simulink model "ProgrammablePulseGenerator"  (Simulink 7.8)
settings: Solver=FixedStepDiscrete  StartTime=0.0  StopTime=10  FixedStep=0.0001  RelTol=1e-3
PostLoadFcn:
  | , if any(exist('dsrtsu_mdlpostloadfcn', 'file') == [2, 3, 6]), try dsrtsu_mdlpostloadfcn('Execute', bdroot); catch fprintf('Error in PostLoadFcn (dsrtsu_mdlpostloadfcn) for model "%s":\n %s\n', bdroot, lasterr); end, end,
settings Model: DSRTSU_INTERNAL_RTI_VER=360  DSRTSU_INTERNAL_RTI_TYPE=rti1104  Creator=kazmionix  LastModifiedBy=kazmionix  BufferReuse=off
settings OptimizationCC: BlockReduction=off  OptimizeBlockIOStorage=off  BufferReuse=off  ExpressionFolding=off  LocalBlockOutputs=off
settings DebuggingCC: FcnCallInpInsideContextMsg=Use local settings  StrictBusMsg=Warning
settings HardwareCC: ProdIntDivRoundTo=Zero  ProdEndianess=BigEndian  ProdHWDeviceType=Generic->Custom  TargetIntDivRoundTo=Zero  TargetEndianess=BigEndian  TargetHWDeviceType=Generic->Custom
settings SFSimCC: SimParseCustomCode=off
settings RTWCC: SystemTargetFile=rti1104.tlc  MakeCommand=make_rti  TemplateMakefile=rti1104.tmf  Description=dSPACE DS1104 Hardware Platform  ProcessScript=rti1104_make_rtw_hook
settings STFCustomTargetCC: ParMdlRefBuildCompliant=on  SystemTargetFile=rti1104.tlc
settings GRTTargetCC: CompOptLevelCompliant=off  ConcurrentExecutionCompliant=off  MatFileLogging=off  ExtModeMexFile=noextcomm
settings CustomProperty: DataType=RTWOptions_EnumType_C__dSPACE_matlab_rti1104_tlc_rti1104_1InitialSimState  Value=RUN
settings EnumStrPairs: String=RUN

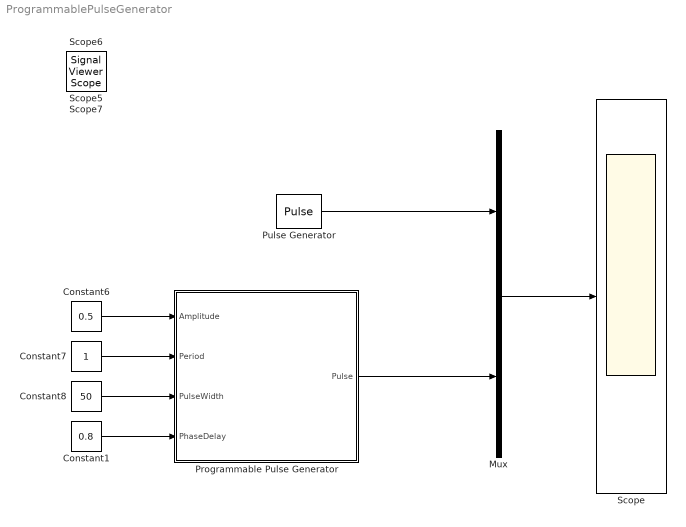
== system ProgrammablePulseGenerator ==
  Constant1 : Constant  Value=0.8
  Constant6 : Constant  Value=0.5
  Constant7 : Constant
  Constant8 : Constant  Value=50
  Mux : Mux  Inputs=2
  Programmable Pulse Generator : Subsystem
  Pulse Generator : DiscretePulseGenerator  PulseType=Time based  Amplitude=0.5  Period=1  PulseWidth=50  PhaseDelay=0.8
  Scope : Scope
      settings: YMin=-1  YMax=1
  Scope5 : SignalViewerScope  IOType=viewer  ZoomMode=xonly  RefreshTime=0.035000
      settings: YMin=0  YMax=2
  Scope6 : SignalViewerScope  IOType=viewer  ZoomMode=yonly  RefreshTime=0.035000
  Scope7 : SignalViewerScope  IOType=viewer  RefreshTime=0.035000
      settings: SaveName=ScopeData2
  wires:
  Constant6/1 -> Programmable Pulse Generator/1(Amplitude)
  Constant7/1 -> Programmable Pulse Generator/2(Period)
  Constant8/1 -> Programmable Pulse Generator/3(PulseWidth)
  Constant1/1 -> Programmable Pulse Generator/4(PhaseDelay)
  Mux/1 -> Scope/1
  Pulse Generator/1 -> Mux/1
  Programmable Pulse Generator/1(Pulse) -> Mux/2

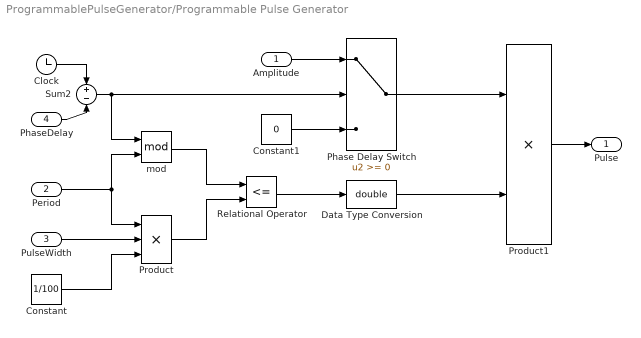
== system ProgrammablePulseGenerator/Programmable Pulse Generator ==
  Amplitude : Inport
  Period : Inport  Port=2
  PulseWidth : Inport  Port=3
  PhaseDelay : Inport  Port=4
  Clock : Clock
  Constant : Constant  Value=1/100
  Constant1 : Constant  Value=0
  Data Type Conversion : DataTypeConversion  OutDataTypeStr=double
  Phase Delay Switch : Switch
  Product : Product  Inputs=3  RndMeth=Zero
  Product1 : Product  RndMeth=Zero
  Relational Operator : RelationalOperator  Operator=<=
  Sum2 : Sum  Inputs=+-
  mod : Math  Operator=mod  SaturateOnIntegerOverflow=on
  Pulse : Outport
  wires:
  Product/1 -> Relational Operator/2
  Product1/1 -> Pulse/1
  Data Type Conversion/1 -> Product1/2
  Relational Operator/1 -> Data Type Conversion/1
  Constant/1 -> Product/3
  PulseWidth/1 -> Product/2
  mod/1 -> Relational Operator/1
  Period/1 -> Product/1, mod/2
  Clock/1 -> Sum2/1
  PhaseDelay/1 -> Sum2/2
  Sum2/1 -> mod/1, Phase Delay Switch/2
  Amplitude/1 -> Phase Delay Switch/1
  Constant1/1 -> Phase Delay Switch/3
  Phase Delay Switch/1 -> Product1/1
